simulink model "DroneControllerCollisionAvoidance"  (R2017a)
settings: Solver=FixedStepAuto  StartTime=0.0  StopTime=t_end  FixedStep=dt  RelTol=1e-3
model workspace (MAT data in the model file):
  SL_ROS_VariableLengthArrays_MaxSizes.CommonInfo.ArrayTruncateAction = 'EmitWarning'
  SL_ROS_VariableLengthArrays_MaxSizes.MsgTypeMap = containers.Map
  SL_ROS_VariableLengthArrays_MaxSizes.MsgTypeMap.serialization.keys = {'sensor_msgs/LaserScan'}
  SL_ROS_VariableLengthArrays_MaxSizes.MsgTypeMap.serialization.values{1}(1).PropertyName = 'Intensities'
  SL_ROS_VariableLengthArrays_MaxSizes.MsgTypeMap.serialization.values{1}(1).DataType = 'single'
  SL_ROS_VariableLengthArrays_MaxSizes.MsgTypeMap.serialization.values{1}(1).MaxLength = 2048
  SL_ROS_VariableLengthArrays_MaxSizes.MsgTypeMap.serialization.values{1}(2).PropertyName = 'Ranges'
  SL_ROS_VariableLengthArrays_MaxSizes.MsgTypeMap.serialization.values{1}(2).DataType = 'single'
  SL_ROS_VariableLengthArrays_MaxSizes.MsgTypeMap.serialization.values{1}(2).MaxLength = 2048
  SL_ROS_VariableLengthArrays_MaxSizes.MsgTypeMap.serialization.uniformity = 0
  SL_ROS_VariableLengthArrays_MaxSizes.MsgTypeMap.serialization.keyType = 'char'
  SL_ROS_VariableLengthArrays_MaxSizes.MsgTypeMap.serialization.valueType = 'any'
values from neighbouring files (symbols this model uses):
  dt = 1/100    (= 0.01)    [startingController.m]
  H_Drone = zeros(5,12)    [startingController.m]
  H_TWB = zeros(3,12)    [startingController.m]
  k1 = a    (= 1)    [startingController.m]
  k10 = a    (= 1)    [startingController.m]
  k11 = a    (= 1)    [startingController.m]
  k12 = a    (= 1)    [startingController.m]
  k2 = a    (= 1)    [startingController.m]
  k3 = a    (= 1)    [startingController.m]
  k4 = a    (= 1)    [startingController.m]
  k5 = a    (= 1)    [startingController.m]
  k6 = a    (= 1)    [startingController.m]
  k7 = a    (= 1)    [startingController.m]
  k8 = a    (= 1)    [startingController.m]
  k9 = a    (= 1)    [startingController.m]
  kd1 = d    (= 0.01)    [startingController.m]
  kd2 = d    (= 0.01)    [startingController.m]
  kd3 = d    (= 0.01)    [startingController.m]
  kd4 = d    (= 0.01)    [startingController.m]
  kp1 = p    (= 10)    [startingController.m]
  kp2 = p    (= 10)    [startingController.m]
  kp3 = p    (= 10)    [startingController.m]
  kp4 = p    (= 10)    [startingController.m]
undefined symbols (not defined in the file or in its folder): Angular, Linear
libraries: robotlib x5, simulink x4, sharedTrackingLibrary x1
settings Model: Creator=Schalker  LastModifiedBy=Schalker

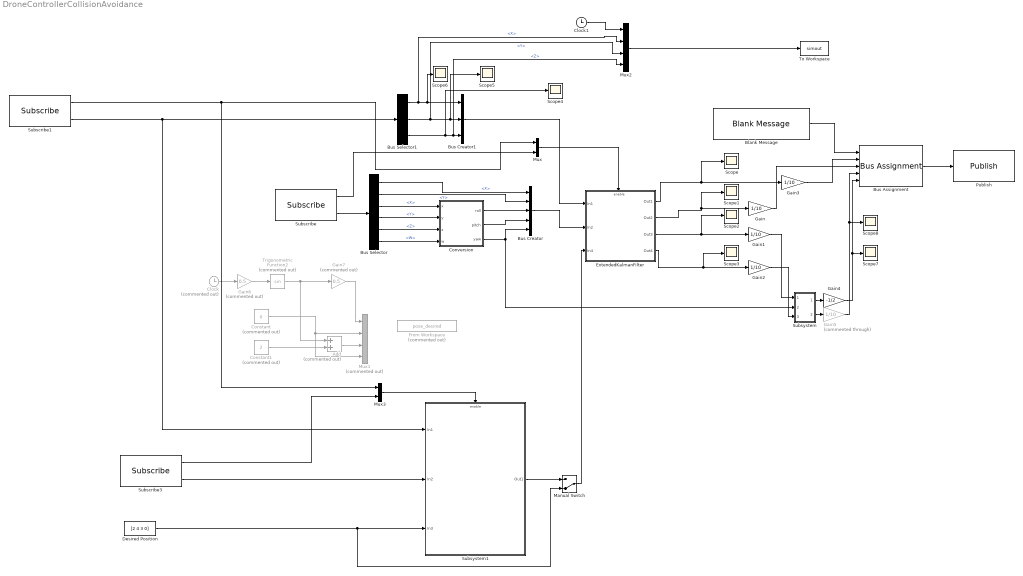
== system DroneControllerCollisionAvoidance ==
  Add : Sum  Commented=on
  Blank Message : robotlib/Blank Message  SourceLibraryInfo=This block requires Robotics System Toolbox  messageType=geometry_msgs/Twist  SampleTime=inf
      settings: SourceProductBaseCode=RO
  Bus Assignment : BusAssignment  AssignedSignals=Linear.Z,Angular.Z,Linear.X,Linear.Y
  Bus Creator : BusCreator  Inputs=5
  Bus Creator1 : BusCreator  Inputs=3
  Bus Selector : BusSelector  OutputSignals=LinearAcceleration.X,LinearAcceleration.Y,Orientation.X,Orientation.Y,Orientation.Z,Orientation.W
  Bus Selector1 : BusSelector  OutputSignals=Pose.Pose.Position.X,Pose.Pose.Position.Y,Pose.Pose.Position.Z
  Clock : Clock  Commented=on
  Clock1 : Clock
  Constant : Constant  Commented=on  Value=0
  Constant1 : Constant  Commented=on  Value=2
  Conversion : MATLAB Function  TreatAsAtomicUnit=on
  Desired Position : Constant  Value=[2 4 3 0]  VectorParams1D=off
  "ExtendedKalmanFilter " : Subsystem
  From Workspace : FromWorkspace  Commented=on  VariableName=pose_desired  OutDataTypeStr=double  SampleTime=0
  Gain{,1..3} (4 alike) : Gain  Gain=1/10
  Gain4 : Gain  Gain=-1/2
  Gain5 : Gain  Commented=through  Gain=1/10
  Gain6 : Gain  Commented=on  Gain=0.5
  Gain7 : Gain  Commented=on  Gain=0.5
  Manual Switch : ManualSwitch  CurrentSetting=0
  Mux : Mux  Inputs=2
  Mux1 : Mux  Commented=on
  Mux2 : Mux
  Mux3 : Mux  Inputs=2
  Publish : robotlib/Publish  SourceLibraryInfo=This block requires Robotics System Toolbox  topicSource=Specify your own  topic=/cmd_vel  messageType=geometry_msgs/Twist  messageQueueLength=1
      settings: SourceProductBaseCode=RO
  Scope{,1..8} (9 alike) : Scope
  Subscribe : robotlib/Subscribe  SourceLibraryInfo=This block requires Robotics System Toolbox  topicSource=Specify your own  topic=/raw_imu  messageType=sensor_msgs/Imu  sampleTime=-1  messageQueueLength=1
      settings: SourceProductBaseCode=RO
  Subscribe1 : robotlib/Subscribe  SourceLibraryInfo=This block requires Robotics System Toolbox  topicSource=Specify your own  topic=/ground_truth/state  messageType=nav_msgs/Odometry  sampleTime=-1  messageQueueLength=1
      settings: SourceProductBaseCode=RO
  Subscribe3 : robotlib/Subscribe  SourceLibraryInfo=This block requires Robotics System Toolbox  topicSource=Select from ROS network  topic=/scan  messageType=sensor_msgs/LaserScan  sampleTime=-1  messageQueueLength=1
      settings: SourceProductBaseCode=RO
  Subsystem : Subsystem
  Subsystem1 : Subsystem
  To Workspace : ToWorkspace  VariableName=simout  SampleTime=-1
      settings: Save2DSignal=2-D array (concatenate along first dimension)
  Trigonometric Function2 : Trigonometry  Commented=on
  wires:
  Blank Message/1 -> Bus Assignment/1
  Bus Assignment/1 -> Publish/1
  "ExtendedKalmanFilter "/2(Out2) -> Scope1/1, Gain/1
  Subscribe/2 -> Bus Selector/1
  Bus Selector/3 -> Conversion/1(x)  "<X>"
  Bus Selector/4 -> Conversion/2(y)  "<Y>"
  Bus Selector/5 -> Conversion/3(z)  "<Z>"
  Bus Selector/6 -> Conversion/4(w)  "<W>"
  Conversion/3(yaw) -> Subsystem/2(In2), Bus Creator/5
  Conversion/2(pitch) -> Bus Creator/4
  Conversion/1(roll) -> Bus Creator/3
  Bus Selector/2 -> Bus Creator/2  "<Y>"
  Bus Selector/1 -> Bus Creator/1  "<X>"
  Bus Creator/1 -> "ExtendedKalmanFilter "/2(In2)
  Bus Selector1/2 -> Scope5/1, Bus Creator1/2, Mux2/3  "<Y>"
  Bus Selector1/3 -> Scope4/1, Mux2/4, Bus Creator1/3  "<Z>"
  Bus Selector1/1 -> Mux2/2, Scope6/1, Bus Creator1/1  "<X>"
  Bus Creator1/1 -> "ExtendedKalmanFilter "/1(In1)
  Mux/1 -> "ExtendedKalmanFilter "/Enable
  Subscribe/1 -> Mux/2
  "ExtendedKalmanFilter "/1(Out1) -> Scope/1, Gain3/1
  "ExtendedKalmanFilter "/4(Out4) -> Scope3/1, Gain2/1
  "ExtendedKalmanFilter "/3(Out3) -> Scope2/1, Gain1/1
  Gain/1 -> Bus Assignment/3
  Gain3/1 -> Bus Assignment/2
  Gain1/1 -> Subsystem/1(In1)
  Gain2/1 -> Subsystem/3(In3)
  Subsystem/1(Out1) -> Gain4/1
  Gain5/1 -> Bus Assignment/4, Scope8/1
  Gain4/1 -> Bus Assignment/5, Scope7/1
  Subsystem/2(Out2) -> Gain5/1
  Clock/1 -> Gain6/1
  Gain6/1 -> Trigonometric Function2/1
  Constant/1 -> Mux1/4, Mux1/2
  Gain7/1 -> Mux1/1
  Trigonometric Function2/1 -> Add/1, Gain7/1
  Add/1 -> Mux1/3
  Constant1/1 -> Add/2
  Clock1/1 -> Mux2/1
  Mux2/1 -> To Workspace/1
  Subscribe1/2 -> Subsystem1/1(In1), Bus Selector1/1
  Subscribe3/2 -> Subsystem1/2(In2)
  Desired Position/1 -> Manual Switch/2, Subsystem1/3(In3)
  Manual Switch/1 -> "ExtendedKalmanFilter "/3(In4)
  Subscribe3/1 -> Mux3/2
  Subscribe1/1 -> Mux3/1, Mux/1
  Mux3/1 -> Subsystem1/Enable
  Subsystem1/1(Out1) -> Manual Switch/1

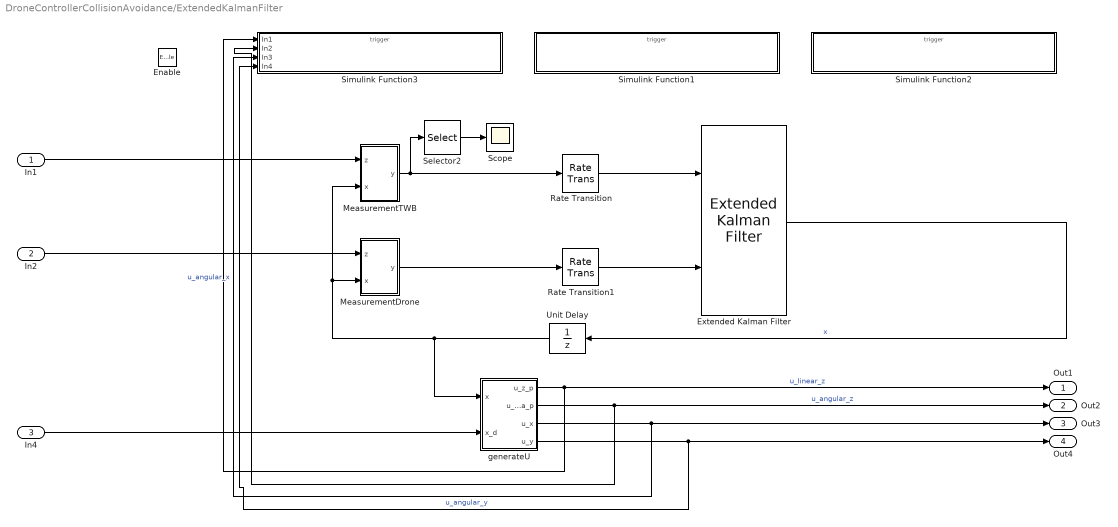
== system DroneControllerCollisionAvoidance/ExtendedKalmanFilter  ==
  In1 : Inport
  In2 : Inport  Port=2
  In4 : Inport  Port=3
  Enable : EnablePort
  Extended Kalman Filter : sharedTrackingLibrary/Extended Kalman Filter  StateTransitionFcn=stateTransitionFcn  HasStateTransitionJacobianFcn=off  HasAdditiveProcessNoise=Additive  ProcessNoise=processNoiseCovariance  HasTimeVaryingProcessNoise=off  HasStateTransitionFcnExtraArgument=0  InitialState=zeros(12, 1)  InitialStateCovariance=10  MeasurementFcn1=measurementTWBFcn  HasMeasurementJacobianFcn1=off  HasMeasurementEnablePort1=off  HasAdditiveMeasurementNoise1=Additive  MeasurementNoise1=measurementNoiseCovarianceTWB  HasTimeVaryingMeasurementNoise1=off  HasMeasurementFcnExtraArgument1=0  MeasurementFcn2=measurementDroneFcn  HasMeasurementJacobianFcn2=off  HasMeasurementEnablePort2=off  HasAdditiveMeasurementNoise2=Additive  MeasurementNoise2=measurementNoiseCovarianceDrone  HasTimeVaryingMeasurementNoise2=off  HasMeasurementFcnExtraArgument2=0  MeasurementFcn3=myMeasurementFcn  HasMeasurementJacobianFcn3=off  HasMeasurementEnablePort3=off  HasAdditiveMeasurementNoise3=Additive  MeasurementNoise3=1  HasTimeVaryingMeasurementNoise3=off  HasMeasurementFcnExtraArgument3=0  MeasurementFcn4=myMeasurementFcn  HasMeasurementJacobianFcn4=off  HasMeasurementEnablePort4=off  HasAdditiveMeasurementNoise4=Additive  MeasurementNoise4=1  HasTimeVaryingMeasurementNoise4=off  HasMeasurementFcnExtraArgument4=0  MeasurementFcn5=myMeasurementFcn  HasMeasurementJacobianFcn5=off  HasMeasurementEnablePort5=off  HasAdditiveMeasurementNoise5=Additive  MeasurementNoise5=1  HasTimeVaryingMeasurementNoise5=off  HasMeasurementFcnExtraArgument5=0  EnableMultirate=on  StateTransitionFcnSampleTime=dt  MeasurementFcn1SampleTime=dt  MeasurementFcn2SampleTime=dt  MeasurementFcn3SampleTime=1  MeasurementFcn4SampleTime=1  MeasurementFcn5SampleTime=1  UseCurrentEstimator=on  OutputStateCovariance=off  DataType=double  SampleTime=1  NumberOfMeasurements=2
  MeasurementDrone : Subsystem
  MeasurementTWB : Subsystem
  Rate Transition : RateTransition
  Rate Transition1 : RateTransition
  Scope : Scope
  Selector2 : Selector  InputPortWidth=3  IndexOptions=Index vector (dialog)  Indices=[3]  OutputSizes=1
  Simulink Function1 : Subsystem  TreatAsAtomicUnit=on
  Simulink Function2 : Subsystem  TreatAsAtomicUnit=on
  Simulink Function3 : Subsystem  TreatAsAtomicUnit=on
  Unit Delay : UnitDelay  SampleTime=-1
  generateU : Subsystem
  Out1 : Outport  OutDataTypeStr=double
  Out2 : Outport  Port=2  OutDataTypeStr=double
  Out3 : Outport  Port=3  OutDataTypeStr=double
  Out4 : Outport  Port=4  OutDataTypeStr=double
  wires:
  In1/1 -> MeasurementTWB/1(z)
  In4/1 -> generateU/2("x_d ")
  Extended Kalman Filter/1 -> Unit Delay/1  "x"
  MeasurementDrone/1(y) -> Rate Transition1/1
  Rate Transition1/1 -> Extended Kalman Filter/2
  In2/1 -> MeasurementDrone/1(z)
  Rate Transition/1 -> Extended Kalman Filter/1
  Unit Delay/1 -> MeasurementDrone/2(x), MeasurementTWB/2(x), generateU/1(x)
  generateU/1(u_z_p) -> Simulink Function3/1(In1), Out1/1  "u_linear_z"
  generateU/4(u_y) -> Simulink Function3/4(In4), Out4/1  "u_angular_y"
  generateU/2(u_theta_p) -> Simulink Function3/2(In2), Out2/1  "u_angular_z"
  generateU/3(u_x) -> Simulink Function3/3(In3), Out3/1  "u_angular_x"
  Selector2/1 -> Scope/1
  MeasurementTWB/1(y) -> Selector2/1, Rate Transition/1

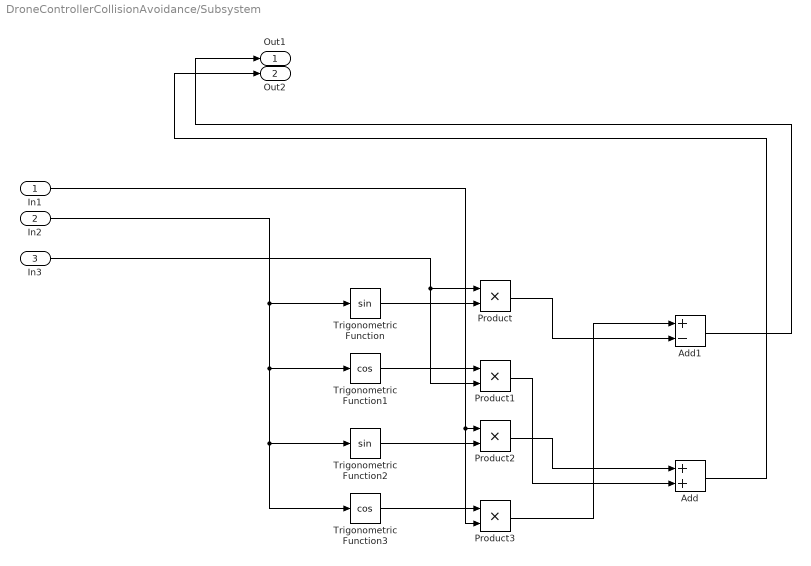
== system DroneControllerCollisionAvoidance/Subsystem ==
  In1 : Inport
  In2 : Inport  Port=2
  In3 : Inport  Port=3
  Add : Sum
  Add1 : Sum  Inputs=+-
  Product{,1..3} (4 alike) : Product
  Trigonometric Function : Trigonometry
  Trigonometric Function1 : Trigonometry  Operator=cos
  Trigonometric Function2 : Trigonometry
  Trigonometric Function3 : Trigonometry  Operator=cos
  Out1 : Outport
  Out2 : Outport  Port=2
  wires:
  Trigonometric Function/1 -> Product/2
  Product/1 -> Add1/2
  Product1/1 -> Add/2
  Add1/1 -> Out1/1
  Product3/1 -> Add1/1
  Add/1 -> Out2/1
  Product2/1 -> Add/1
  Trigonometric Function1/1 -> Product1/1
  In1/1 -> Product3/2, Product2/1
  In2/1 -> Trigonometric Function3/1, Trigonometric Function2/1, Trigonometric Function1/1, Trigonometric Function/1
  Trigonometric Function3/1 -> Product3/1
  Trigonometric Function2/1 -> Product2/2
  In3/1 -> Product1/2, Product/1

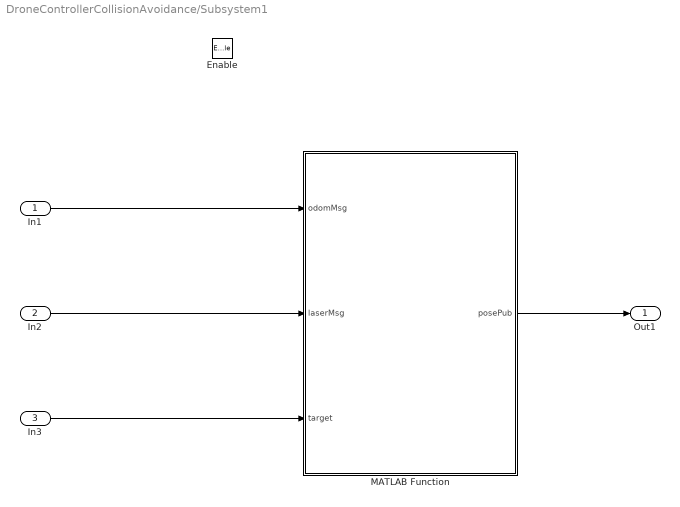
== system DroneControllerCollisionAvoidance/Subsystem1 ==
  In1 : Inport
  In2 : Inport  Port=2
  In3 : Inport  Port=3
  Enable : EnablePort
  MATLAB Function : MATLAB Function  TreatAsAtomicUnit=on
  Out1 : Outport
  wires:
  MATLAB Function/1(posePub) -> Out1/1
  In2/1 -> MATLAB Function/2(laserMsg)
  In1/1 -> MATLAB Function/1(odomMsg)
  In3/1 -> MATLAB Function/3(target)

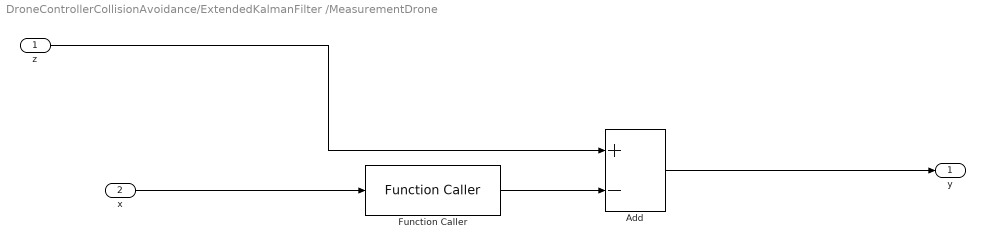
== system DroneControllerCollisionAvoidance/ExtendedKalmanFilter /MeasurementDrone ==
  z : Inport
  x : Inport  Port=2
  Add : Sum  Inputs=+-
  Function Caller : FunctionCaller  FunctionPrototype=y = measurementDroneFcn(x)
  y : Outport
  wires:
  Function Caller/1 -> Add/2
  x/1 -> Function Caller/1
  z/1 -> Add/1
  Add/1 -> y/1

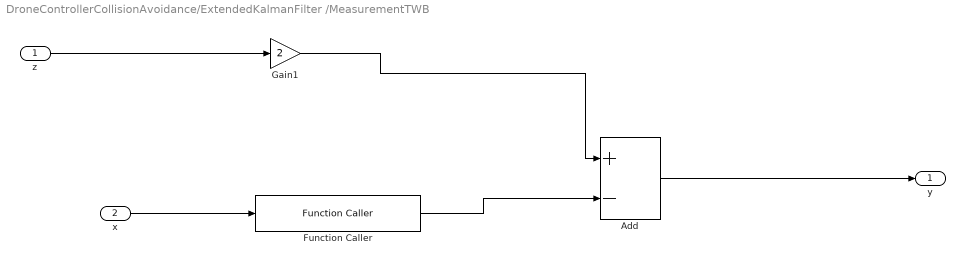
== system DroneControllerCollisionAvoidance/ExtendedKalmanFilter /MeasurementTWB ==
  z : Inport
  x : Inport  Port=2
  Add : Sum  Inputs=+-
  Function Caller : FunctionCaller  FunctionPrototype=y = measurementTWBFcn(x)
  Gain1 : Gain  Gain=2
  y : Outport
  wires:
  z/1 -> Gain1/1
  Add/1 -> y/1
  Function Caller/1 -> Add/2
  x/1 -> Function Caller/1
  Gain1/1 -> Add/1

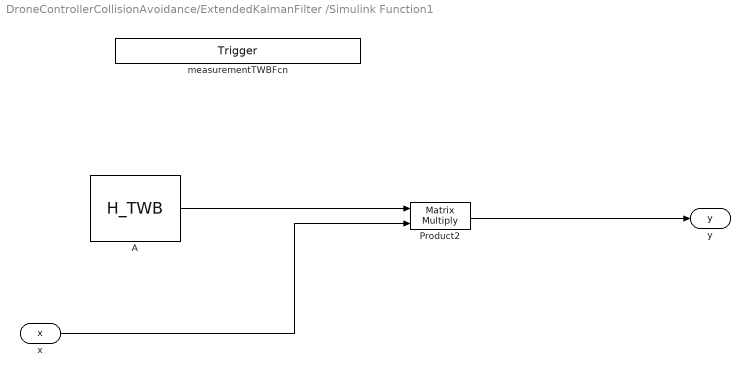
== system DroneControllerCollisionAvoidance/ExtendedKalmanFilter /Simulink Function1 ==
  measurementTWBFcn : TriggerPort  TriggerType=function-call  IsSimulinkFunction=on  FunctionName=measurementTWBFcn  VariantControl=Variant
  A : Constant  Value=H_TWB
  Product2 : Product  Multiplication=Matrix(*)
  x : ArgIn  DisableCoverage=on  PortDimensions=12  ArgumentName=x
  y : ArgOut  DisableCoverage=on  PortDimensions=3  ArgumentName=y
  wires:
  A/1 -> Product2/1
  x/1 -> Product2/2
  Product2/1 -> y/1

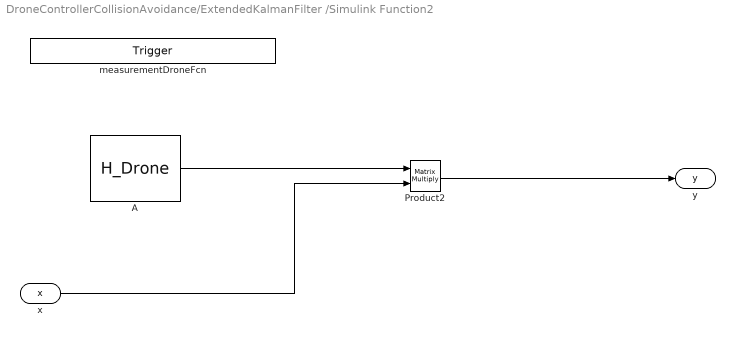
== system DroneControllerCollisionAvoidance/ExtendedKalmanFilter /Simulink Function2 ==
  measurementDroneFcn : TriggerPort  TriggerType=function-call  IsSimulinkFunction=on  FunctionName=measurementDroneFcn  VariantControl=Variant
  A : Constant  Value=H_Drone
  Product2 : Product  Multiplication=Matrix(*)
  x : ArgIn  DisableCoverage=on  PortDimensions=12  ArgumentName=x
  y : ArgOut  DisableCoverage=on  PortDimensions=5  ArgumentName=y
  wires:
  Product2/1 -> y/1
  A/1 -> Product2/1
  x/1 -> Product2/2

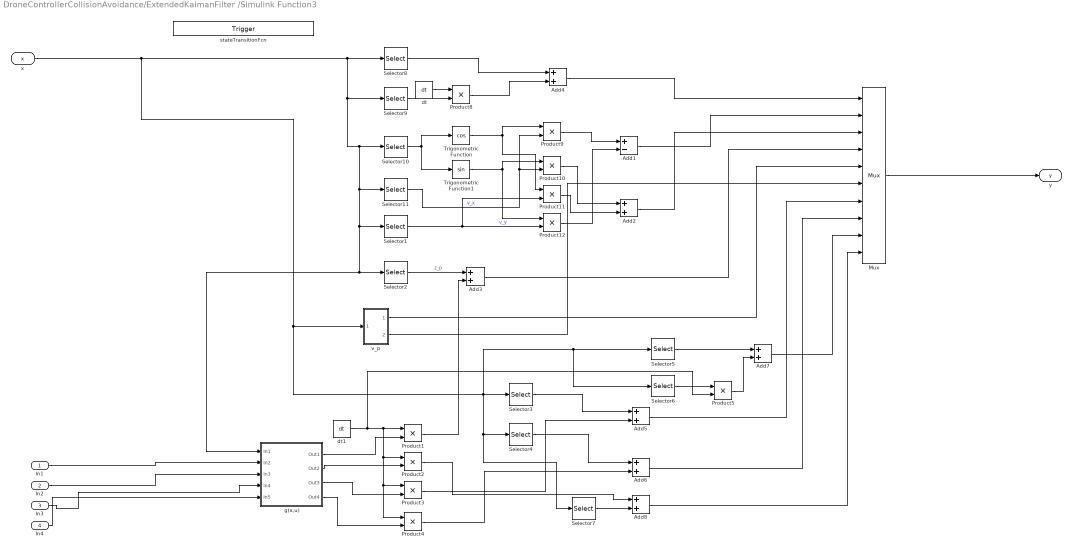
== system DroneControllerCollisionAvoidance/ExtendedKalmanFilter /Simulink Function3 ==
  In1 : Inport
  In2 : Inport  Port=2
  In3 : Inport  Port=3
  In4 : Inport  Port=4
  stateTransitionFcn : TriggerPort  TriggerType=function-call  IsSimulinkFunction=on  FunctionName=stateTransitionFcn  VariantControl=Variant
  Add1 : Sum  Inputs=+-
  Add{2..8} (7 alike) : Sum
  Mux : Mux  Inputs=10
  Product{1..5,8..12} (10 alike) : Product
  Selector1 : Selector  InputPortWidth=12  IndexOptions=Index vector (dialog)  Indices=[8]  OutputSizes=1
  Selector10 : Selector  InputPortWidth=12  IndexOptions=Index vector (dialog)  Indices=[11]  OutputSizes=1
  Selector11 : Selector  InputPortWidth=12  IndexOptions=Index vector (dialog)  Indices=[7]  OutputSizes=1
  Selector2 : Selector  InputPortWidth=12  IndexOptions=Index vector (dialog)  Indices=[6]  OutputSizes=1
  Selector3 : Selector  InputPortWidth=12  IndexOptions=Index vector (dialog)  Indices=[9]  OutputSizes=1
  Selector4 : Selector  InputPortWidth=12  IndexOptions=Index vector (dialog)  Indices=[10]  OutputSizes=1
  Selector5 : Selector  InputPortWidth=12  IndexOptions=Index vector (dialog)  Indices=[11]  OutputSizes=1
  Selector6 : Selector  InputPortWidth=12  IndexOptions=Index vector (dialog)  Indices=[12]  OutputSizes=1
  Selector7 : Selector  InputPortWidth=12  IndexOptions=Index vector (dialog)  Indices=[12]  OutputSizes=1
  Selector8 : Selector  InputPortWidth=12  IndexOptions=Index vector (dialog)  Indices=[1 2 3]  OutputSizes=1
  Selector9 : Selector  InputPortWidth=12  IndexOptions=Index vector (dialog)  Indices=[4 5 6]  OutputSizes=1
  Trigonometric Function : Trigonometry  Operator=cos
  Trigonometric Function1 : Trigonometry
  dt : Constant  Value=dt
  dt1 : Constant  Value=dt
  g(x,u) : Subsystem
  v_p : Subsystem
  x : ArgIn  DisableCoverage=on  PortDimensions=12  ArgumentName=x
  y : ArgOut  DisableCoverage=on  PortDimensions=12  ArgumentName=y
  wires:
  x/1 -> Selector6/1, Selector5/1, Selector7/1, Selector4/1, Selector3/1, v_p/1(In1), Selector8/1, Selector11/1, Selector1/1, Selector2/1, g(x,u)/1(In1), Selector10/1, Selector9/1
  Selector9/1 -> Product8/2
  dt/1 -> Product8/1
  Product8/1 -> Add4/2
  Selector8/1 -> Add4/1
  Add4/1 -> Mux/1
  Selector10/1 -> Trigonometric Function1/1, Trigonometric Function/1
  Trigonometric Function/1 -> Product11/1, Product9/1
  Trigonometric Function1/1 -> Product12/1, Product10/1
  In1/1 -> g(x,u)/2(In2)
  Selector11/1 -> Product10/2, Product9/2  "v_x"
  Selector1/1 -> Product12/2, Product11/2  "v_y"
  Product9/1 -> Add1/1
  Product12/1 -> Add1/2
  Product10/1 -> Add2/1
  Product11/1 -> Add2/2
  Selector2/1 -> Add3/1  "z_p"
  g(x,u)/1(Out1) -> Product1/2
  Product1/1 -> Add3/2
  g(x,u)/2(Out2) -> Product2/2
  g(x,u)/3(Out3) -> Product3/2
  g(x,u)/4(Out4) -> Product4/2
  Add3/1 -> Mux/4
  v_p/1(Out1) -> Mux/5
  v_p/2(Out2) -> Mux/6
  Add1/1 -> Mux/2
  Add2/1 -> Mux/3
  Selector3/1 -> Add5/1
  Product3/1 -> Add5/2
  Selector4/1 -> Add6/1
  Product4/1 -> Add6/2
  Add5/1 -> Mux/7
  Add6/1 -> Mux/8
  Selector6/1 -> Product5/1
  dt1/1 -> Product5/2, Product2/1, Product4/1, Product3/1, Product1/1
  Selector5/1 -> Add7/1
  Product5/1 -> Add7/2
  Add7/1 -> Mux/9
  Selector7/1 -> Add8/2
  Product2/1 -> Add8/1
  Add8/1 -> Mux/10
  Mux/1 -> y/1
  In2/1 -> g(x,u)/3(In3)
  In3/1 -> g(x,u)/4(In4)
  In4/1 -> g(x,u)/5(In5)

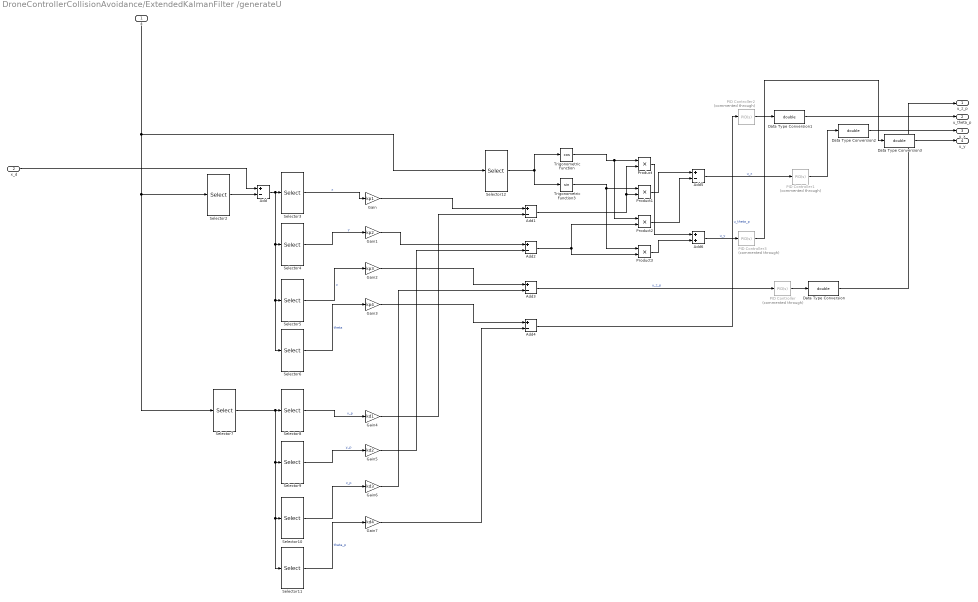
== system DroneControllerCollisionAvoidance/ExtendedKalmanFilter /generateU ==
  x : Inport
  "x_d " : Inport  Port=2
  Add{,1..5} (6 alike) : Sum  Inputs=+-
  Add6 : Sum
  Data Type Conversion{,1..3} (4 alike) : DataTypeConversion  OutDataTypeStr=double
  Gain : Gain  Gain=kp1
  Gain1 : Gain  Gain=kp2
  Gain2 : Gain  Gain=kp3
  Gain3 : Gain  Gain=kp4
  Gain4 : Gain  Gain=kd1
  Gain5 : Gain  Gain=kd2
  Gain6 : Gain  Gain=kd3
  Gain7 : Gain  Gain=kd4
  PID Controller : simulink/Continuous/PID Controller  Commented=through  Controller=PID  TimeDomain=Continuous-time  SampleTime=-1  IntegratorMethod=Forward Euler  FilterMethod=Forward Euler  Form=Parallel  UseFilter=on  ControllerParametersSource=internal  P=1  I=10  D=0  N=100  InitialConditionSource=internal  InitialConditionForIntegrator=0  InitialConditionForFilter=0  ExternalReset=none  LimitOutput=off  UpperSaturationLimit=inf  LowerSaturationLimit=-inf  LinearizeAsGain=on  AntiWindupMode=none  Kb=1  TrackingMode=off  Kt=1  PParamMin=[]  PParamMax=[]  IParamMin=[]  IParamMax=[]  DParamMin=[]  DParamMax=[]  NParamMin=[]  NParamMax=[]  KbParamMin=[]  KbParamMax=[]  KtParamMin=[]  KtParamMax=[]  POutMin=[]  POutMax=[]  IOutMin=[]  IOutMax=[]  DOutMin=[]  DOutMax=[]  NOutMin=[]  NOutMax=[]  KbOutMin=[]  KbOutMax=[]  KtOutMin=[]  KtOutMax=[]  IntegratorOutMin=[]  IntegratorOutMax=[]  FilterOutMin=[]  FilterOutMax=[]  SumOutMin=[]  SumOutMax=[]  SumI1OutMin=[]  SumI1OutMax=[]  SumI2OutMin=[]  SumI2OutMax=[]  SumI3OutMin=[]  SumI3OutMax=[]  SumDOutMin=[]  SumDOutMax=[]  SaturationOutMin=[]  SaturationOutMax=[]  IntegratorContinuousStateAttributes=''  IntegratorStateMustResolveToSignalObject=off  IntegratorRTWStateStorageClass=Auto  FilterContinuousStateAttributes=''  FilterStateMustResolveToSignalObject=off  FilterRTWStateStorageClass=Auto  DifferentiatorICPrevScaledInput=0  DifferentiatorOutMin=[]  DifferentiatorOutMax=[]  InitialConditionSetting=State (most efficient)
  PID Controller1 : simulink/Continuous/PID Controller  Commented=through  Controller=PID  TimeDomain=Continuous-time  SampleTime=-1  IntegratorMethod=Forward Euler  FilterMethod=Forward Euler  Form=Parallel  UseFilter=on  ControllerParametersSource=internal  P=1  I=1  D=0  N=100  InitialConditionSource=internal  InitialConditionForIntegrator=0  InitialConditionForFilter=0  ExternalReset=none  LimitOutput=off  UpperSaturationLimit=inf  LowerSaturationLimit=-inf  LinearizeAsGain=on  AntiWindupMode=none  Kb=1  TrackingMode=off  Kt=1  PParamMin=[]  PParamMax=[]  IParamMin=[]  IParamMax=[]  DParamMin=[]  DParamMax=[]  NParamMin=[]  NParamMax=[]  KbParamMin=[]  KbParamMax=[]  KtParamMin=[]  KtParamMax=[]  POutMin=[]  POutMax=[]  IOutMin=[]  IOutMax=[]  DOutMin=[]  DOutMax=[]  NOutMin=[]  NOutMax=[]  KbOutMin=[]  KbOutMax=[]  KtOutMin=[]  KtOutMax=[]  IntegratorOutMin=[]  IntegratorOutMax=[]  FilterOutMin=[]  FilterOutMax=[]  SumOutMin=[]  SumOutMax=[]  SumI1OutMin=[]  SumI1OutMax=[]  SumI2OutMin=[]  SumI2OutMax=[]  SumI3OutMin=[]  SumI3OutMax=[]  SumDOutMin=[]  SumDOutMax=[]  SaturationOutMin=[]  SaturationOutMax=[]  IntegratorContinuousStateAttributes=''  IntegratorStateMustResolveToSignalObject=off  IntegratorRTWStateStorageClass=Auto  FilterContinuousStateAttributes=''  FilterStateMustResolveToSignalObject=off  FilterRTWStateStorageClass=Auto  DifferentiatorICPrevScaledInput=0  DifferentiatorOutMin=[]  DifferentiatorOutMax=[]  InitialConditionSetting=State (most efficient)
  PID Controller2 : simulink/Continuous/PID Controller  Commented=through  Controller=PID  TimeDomain=Continuous-time  SampleTime=-1  IntegratorMethod=Forward Euler  FilterMethod=Forward Euler  Form=Parallel  UseFilter=on  ControllerParametersSource=internal  P=1  I=1  D=0  N=100  InitialConditionSource=internal  InitialConditionForIntegrator=0  InitialConditionForFilter=0  ExternalReset=none  LimitOutput=off  UpperSaturationLimit=inf  LowerSaturationLimit=-inf  LinearizeAsGain=on  AntiWindupMode=none  Kb=1  TrackingMode=off  Kt=1  PParamMin=[]  PParamMax=[]  IParamMin=[]  IParamMax=[]  DParamMin=[]  DParamMax=[]  NParamMin=[]  NParamMax=[]  KbParamMin=[]  KbParamMax=[]  KtParamMin=[]  KtParamMax=[]  POutMin=[]  POutMax=[]  IOutMin=[]  IOutMax=[]  DOutMin=[]  DOutMax=[]  NOutMin=[]  NOutMax=[]  KbOutMin=[]  KbOutMax=[]  KtOutMin=[]  KtOutMax=[]  IntegratorOutMin=[]  IntegratorOutMax=[]  FilterOutMin=[]  FilterOutMax=[]  SumOutMin=[]  SumOutMax=[]  SumI1OutMin=[]  SumI1OutMax=[]  SumI2OutMin=[]  SumI2OutMax=[]  SumI3OutMin=[]  SumI3OutMax=[]  SumDOutMin=[]  SumDOutMax=[]  SaturationOutMin=[]  SaturationOutMax=[]  IntegratorContinuousStateAttributes=''  IntegratorStateMustResolveToSignalObject=off  IntegratorRTWStateStorageClass=Auto  FilterContinuousStateAttributes=''  FilterStateMustResolveToSignalObject=off  FilterRTWStateStorageClass=Auto  DifferentiatorICPrevScaledInput=0  DifferentiatorOutMin=[]  DifferentiatorOutMax=[]  InitialConditionSetting=State (most efficient)
  PID Controller3 : simulink/Continuous/PID Controller  Commented=through  Controller=PID  TimeDomain=Continuous-time  SampleTime=-1  IntegratorMethod=Forward Euler  FilterMethod=Forward Euler  Form=Parallel  UseFilter=on  ControllerParametersSource=internal  P=1  I=1  D=0  N=100  InitialConditionSource=internal  InitialConditionForIntegrator=0  InitialConditionForFilter=0  ExternalReset=none  LimitOutput=off  UpperSaturationLimit=inf  LowerSaturationLimit=-inf  LinearizeAsGain=on  AntiWindupMode=none  Kb=1  TrackingMode=off  Kt=1  PParamMin=[]  PParamMax=[]  IParamMin=[]  IParamMax=[]  DParamMin=[]  DParamMax=[]  NParamMin=[]  NParamMax=[]  KbParamMin=[]  KbParamMax=[]  KtParamMin=[]  KtParamMax=[]  POutMin=[]  POutMax=[]  IOutMin=[]  IOutMax=[]  DOutMin=[]  DOutMax=[]  NOutMin=[]  NOutMax=[]  KbOutMin=[]  KbOutMax=[]  KtOutMin=[]  KtOutMax=[]  IntegratorOutMin=[]  IntegratorOutMax=[]  FilterOutMin=[]  FilterOutMax=[]  SumOutMin=[]  SumOutMax=[]  SumI1OutMin=[]  SumI1OutMax=[]  SumI2OutMin=[]  SumI2OutMax=[]  SumI3OutMin=[]  SumI3OutMax=[]  SumDOutMin=[]  SumDOutMax=[]  SaturationOutMin=[]  SaturationOutMax=[]  IntegratorContinuousStateAttributes=''  IntegratorStateMustResolveToSignalObject=off  IntegratorRTWStateStorageClass=Auto  FilterContinuousStateAttributes=''  FilterStateMustResolveToSignalObject=off  FilterRTWStateStorageClass=Auto  DifferentiatorICPrevScaledInput=0  DifferentiatorOutMin=[]  DifferentiatorOutMax=[]  InitialConditionSetting=State (most efficient)
  Product{,1..3} (4 alike) : Product
  Selector10 : Selector  InputPortWidth=4  IndexOptions=Index vector (dialog)  Indices=3  OutputSizes=1
  Selector11 : Selector  InputPortWidth=4  IndexOptions=Index vector (dialog)  Indices=4  OutputSizes=1
  Selector12 : Selector  InputPortWidth=12  IndexOptions=Index vector (dialog)  Indices=11  OutputSizes=1
  Selector2 : Selector  InputPortWidth=12  IndexOptions=Index vector (dialog)  Indices=[1 2 3 11]  OutputSizes=1
  Selector3 : Selector  InputPortWidth=4  IndexOptions=Index vector (dialog)  Indices=[1]  OutputSizes=1
  Selector4 : Selector  InputPortWidth=4  IndexOptions=Index vector (dialog)  Indices=2  OutputSizes=1
  Selector5 : Selector  InputPortWidth=4  IndexOptions=Index vector (dialog)  Indices=3  OutputSizes=1
  Selector6 : Selector  InputPortWidth=4  IndexOptions=Index vector (dialog)  Indices=4  OutputSizes=1
  Selector7 : Selector  InputPortWidth=12  IndexOptions=Index vector (dialog)  Indices=[4 5 6 12]  OutputSizes=1
  Selector8 : Selector  InputPortWidth=4  IndexOptions=Index vector (dialog)  Indices=[1]  OutputSizes=1
  Selector9 : Selector  InputPortWidth=4  IndexOptions=Index vector (dialog)  Indices=2  OutputSizes=1
  Trigonometric Function : Trigonometry  Operator=cos
  Trigonometric Function3 : Trigonometry
  u_z_p : Outport
  u_theta_p : Outport  Port=2
  u_x : Outport  Port=3
  u_y : Outport  Port=4
  wires:
  Selector3/1 -> Gain/1  "x"
  "x_d "/1 -> Add/1
  Gain1/1 -> Add2/1
  Product2/1 -> Add5/2
  Add2/1 -> Product3/2, Product2/2
  Selector4/1 -> Gain1/1  "y"
  Add4/1 -> PID Controller2/1  "u_theta_p"
  Selector2/1 -> Add/2
  Add6/1 -> PID Controller3/1  "u_y"
  Add5/1 -> PID Controller1/1  "u_x"
  Product1/1 -> Add5/1
  Gain/1 -> Add1/1
  Selector6/1 -> Gain3/1  "theta"
  Gain7/1 -> Add4/2
  Selector11/1 -> Gain7/1  "theta_p"
  Selector7/1 -> Selector8/1, Selector9/1, Selector10/1, Selector11/1
  Selector10/1 -> Gain6/1  "z_p"
  Selector9/1 -> Gain5/1  "y_p"
  Selector8/1 -> Gain4/1  "x_p"
  Gain6/1 -> Add3/2
  Gain3/1 -> Add4/1
  Add1/1 -> Product1/2, Product/2
  Selector12/1 -> Trigonometric Function/1, Trigonometric Function3/1
  Add/1 -> Selector6/1, Selector5/1, Selector4/1, Selector3/1
  Gain4/1 -> Add1/2
  x/1 -> Selector12/1, Selector7/1, Selector2/1
  Gain2/1 -> Add3/1
  Product3/1 -> Add6/2
  Product/1 -> Add6/1
  Trigonometric Function/1 -> Product2/1, Product/1
  Trigonometric Function3/1 -> Product3/1, Product1/1
  Gain5/1 -> Add2/2
  Add3/1 -> PID Controller/1  "u_z_p"
  Selector5/1 -> Gain2/1  "z"
  Data Type Conversion/1 -> u_z_p/1
  Data Type Conversion1/1 -> u_theta_p/1
  Data Type Conversion2/1 -> u_x/1
  Data Type Conversion3/1 -> u_y/1
  PID Controller/1 -> Data Type Conversion/1
  PID Controller1/1 -> Data Type Conversion2/1
  PID Controller2/1 -> Data Type Conversion1/1
  PID Controller3/1 -> Data Type Conversion3/1

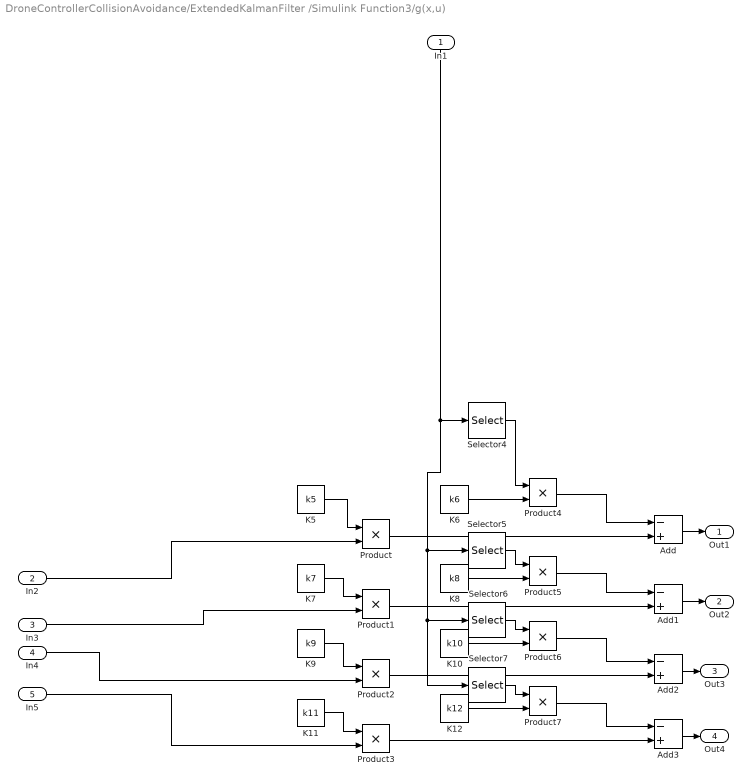
== system DroneControllerCollisionAvoidance/ExtendedKalmanFilter /Simulink Function3/g(x,u) ==
  In1 : Inport
  In2 : Inport  Port=2
  In3 : Inport  Port=3
  In4 : Inport  Port=4
  In5 : Inport  Port=5
  Add{,1..3} (4 alike) : Sum  Inputs=-+
  K10 : Constant  Value=k10
  K11 : Constant  Value=k11
  K12 : Constant  Value=k12
  K5 : Constant  Value=k5
  K6 : Constant  Value=k6
  K7 : Constant  Value=k7
  K8 : Constant  Value=k8
  K9 : Constant  Value=k9
  Product{,1..7} (8 alike) : Product
  Selector4 : Selector  InputPortWidth=12  IndexOptions=Index vector (dialog)  Indices=[6]  OutputSizes=1
  Selector5 : Selector  InputPortWidth=12  IndexOptions=Index vector (dialog)  Indices=[12]  OutputSizes=1
  Selector6 : Selector  InputPortWidth=12  IndexOptions=Index vector (dialog)  Indices=[9]  OutputSizes=1
  Selector7 : Selector  InputPortWidth=12  IndexOptions=Index vector (dialog)  Indices=[10]  OutputSizes=1
  Out1 : Outport
  Out2 : Outport  Port=2
  Out3 : Outport  Port=3
  Out4 : Outport  Port=4
  wires:
  K7/1 -> Product1/1
  Selector6/1 -> Product6/1
  In4/1 -> Product2/2
  Product/1 -> Add/2
  Product6/1 -> Add2/1
  In2/1 -> Product/2
  Add2/1 -> Out3/1
  In1/1 -> Selector7/1, Selector6/1, Selector5/1, Selector4/1
  Add3/1 -> Out4/1
  Add/1 -> Out1/1
  Add1/1 -> Out2/1
  K9/1 -> Product2/1
  Selector4/1 -> Product4/1
  Product2/1 -> Add2/2
  K8/1 -> Product5/2
  Product3/1 -> Add3/2
  Product1/1 -> Add1/2
  Selector5/1 -> Product5/1
  Product5/1 -> Add1/1
  K5/1 -> Product/1
  K12/1 -> Product7/2
  Product7/1 -> Add3/1
  K10/1 -> Product6/2
  Product4/1 -> Add/1
  In3/1 -> Product1/2
  Selector7/1 -> Product7/1
  K11/1 -> Product3/1
  K6/1 -> Product4/2
  In5/1 -> Product3/2

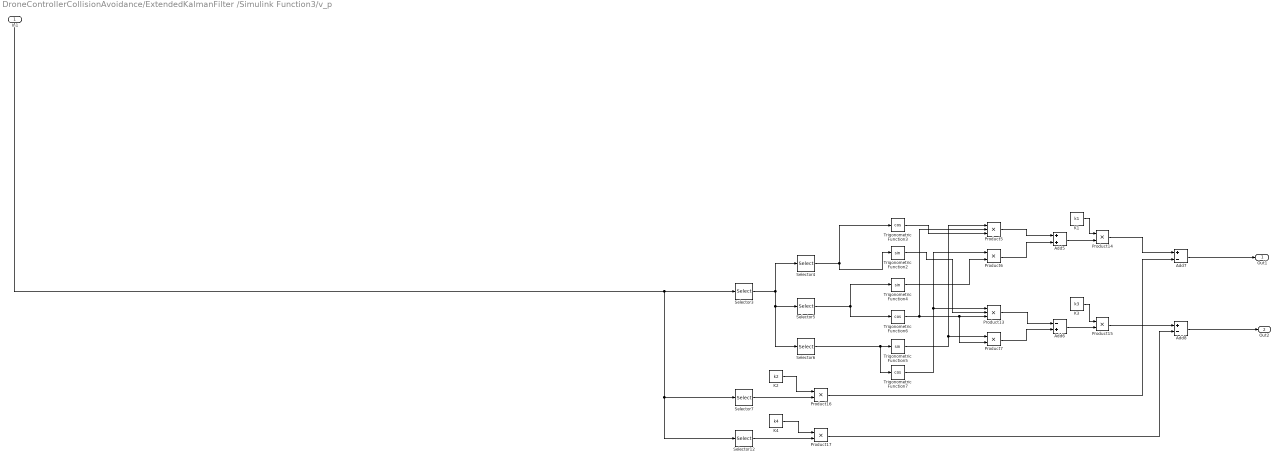
== system DroneControllerCollisionAvoidance/ExtendedKalmanFilter /Simulink Function3/v_p ==
  In1 : Inport
  Add5 : Sum
  Add6 : Sum  Inputs=-+
  Add7 : Sum  Inputs=+-
  Add8 : Sum  Inputs=+-
  K1 : Constant  Value=k1
  K2 : Constant  Value=k2
  K3 : Constant  Value=k3
  K4 : Constant  Value=k4
  Product13 : Product  Inputs=3
  Product{6..7,14..17} (6 alike) : Product
  Product5 : Product  Inputs=3
  Selector12 : Selector  InputPortWidth=12  IndexOptions=Index vector (dialog)  Indices=[8]  OutputSizes=1
  Selector3 : Selector  InputPortWidth=12  IndexOptions=Index vector (dialog)  Indices=[9 10 11]  OutputSizes=1
  Selector4 : Selector  InputPortWidth=3  IndexOptions=Index vector (dialog)  Indices=[1]  OutputSizes=1
  Selector5 : Selector  InputPortWidth=3  IndexOptions=Index vector (dialog)  Indices=[2]  OutputSizes=1
  Selector6 : Selector  InputPortWidth=3  IndexOptions=Index vector (dialog)  Indices=[3]  OutputSizes=1
  Selector7 : Selector  InputPortWidth=12  IndexOptions=Index vector (dialog)  Indices=[7]  OutputSizes=1
  Trigonometric Function2 : Trigonometry
  Trigonometric Function3 : Trigonometry  Operator=cos
  Trigonometric Function4 : Trigonometry
  Trigonometric Function5 : Trigonometry
  Trigonometric Function6 : Trigonometry  Operator=cos
  Trigonometric Function7 : Trigonometry  Operator=cos
  Out1 : Outport
  Out2 : Outport  Port=2
  wires:
  In1/1 -> Selector12/1, Selector7/1, Selector3/1
  Selector6/1 -> Trigonometric Function5/1, Trigonometric Function7/1
  Trigonometric Function4/1 -> Product6/2
  Product6/1 -> Add5/2
  Add7/1 -> Out1/1
  Add5/1 -> Product14/2
  K1/1 -> Product14/1
  Product13/1 -> Add6/1
  Product16/1 -> Add7/2
  Product17/1 -> Add8/2
  Trigonometric Function6/1 -> Product7/2, Product13/3, Product5/2
  K2/1 -> Product16/1
  Selector5/1 -> Trigonometric Function6/1, Trigonometric Function4/1
  Trigonometric Function2/1 -> Product13/2
  Add8/1 -> Out2/1
  Selector7/1 -> Product16/2
  Product14/1 -> Add7/1
  Trigonometric Function5/1 -> Product5/1, Product7/1
  Product5/1 -> Add5/1
  Selector12/1 -> Product17/2
  Selector4/1 -> Trigonometric Function3/1, Trigonometric Function2/1
  Selector3/1 -> Selector6/1, Selector5/1, Selector4/1
  Product7/1 -> Add6/2
  Product15/1 -> Add8/1
  Add6/1 -> Product15/2
  Trigonometric Function7/1 -> Product13/1, Product6/1
  Trigonometric Function3/1 -> Product5/3
  K4/1 -> Product17/1
  K3/1 -> Product15/1

== matlab function DroneControllerCollisionAvoidance/Conversion ==
  data: roll output; pitch output; yaw output; x input; y input; z input; w input
function [roll,pitch,yaw]  = quat2eul(x,y,z,w)
%#codegen

% Convert the quaternion to a yaw angle (zyx euler angle)
eul = quat2eul([w,x,y,z]);
roll = eul(3);
pitch = eul(2);
yaw = eul(1);

end

== matlab function DroneControllerCollisionAvoidance/Subsystem1/MATLAB Function ==
  data: odomMsg input; laserMsg input; posePub output; target input
function posePub = hectorQuadrotorPathPlanningSimulinkFunction(odomMsg, laserMsg, target)
%UNTITLED2 Summary of this function goes here
%   Detailed explanation goes here
posePub = target;
target = target([1:3]);
originTarget = target;
lastPositions = zeros(10,3);
pose = readPose(odomMsg);

if sqrt(sum((pose([1:3]) - target).^2)) > 0.1
    [minDist, data] = findObstacle(laserMsg, pose);
    data = [data(1,:) pose(3)];
    lastPositions = circshift(lastPositions,1);
    lastPositions(1,:) = pose([1:3]);
    v = sqrt(sum((pose([1:3]) - target).^2));
    if v > 1 && sqrt(sum(std(lastPositions).^2)) < 0.075  % abs(sum(F)) < 1
        target(3) = target(3) + 0.5; % * v;
    else
        target = originTarget;
    end
    u = hectorQuadrotorComputePotentialField(target,...
        pose([1:3]), data, minDist);
    posePub = [pose([1:3]) + u, 0];
end
end

function [minDist, dataWorld] = findObstacle(obj, pose)
defaults.RangeLimits = [0.5, obj.RangeMax];
R = obj.Ranges;
validIdx = isfinite(R) & R >= defaults.RangeLimits(1) & R <= defaults.RangeLimits(2);
R = R(validIdx);
minDist = min(R);
validIdx = find(R==minDist);
angles = [obj.AngleMin : obj.AngleIncrement : obj.AngleMax];
cartAngles = angles(validIdx);
x = cos(cartAngles) .* R(validIdx,1);
y = sin(cartAngles) .* R(validIdx,1);
cart = double([x,y]) * [0 1; 1 0];

th = pose(4)-pi/2;
dataWorld = cart*[cos(th) sin(th);-sin(th) cos(th)] ...
    + repmat(pose(1:2),[numel(cart(:,1)),1]);
end

function pose = readPose(odomMsg)
%readPose Extract the robot odometry reading as [x y theta] vector

% Extract the x, y, and theta coordinates
poseMsg = odomMsg.Pose.Pose;
xpos = poseMsg.Position.X;
ypos = poseMsg.Position.Y;
zpos = poseMsg.Position.Z;
quat = poseMsg.Orientation;
angles = quat2eul([quat.W quat.X quat.Y quat.Z]);
theta = angles(1);
pose = [xpos, ypos, zpos, theta];

end
